simulink model "PID_Controller_ref"  (R2020b)
settings: Solver=ode45  StartTime=0.0  StopTime=0.2  RelTol=1e-3
undefined symbols (not defined in the file or in its folder): Kd, Ki, Kp
settings Model: DataDictionary=DataDictionary.sldd  PacingRate=1000000  Creator=abhin  LastModifiedBy=abhin
settings SolverCC: InitialStep=0.0001  AlgebraicLoopSolver=LineSearch
settings DataIOCC: SaveOutput=off  SaveTime=off

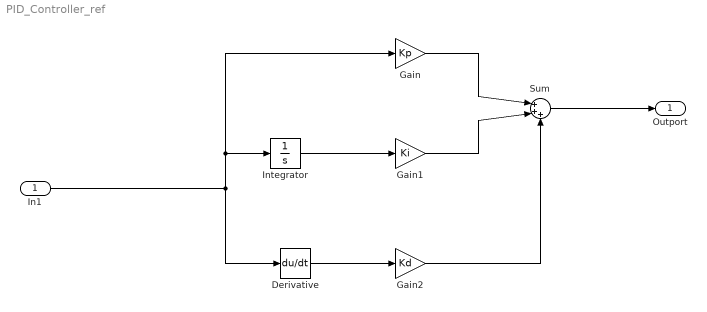
== system PID_Controller_ref ==
  In1 : Inport  OutDataTypeStr=double  PortDimensions=1  SampleTime=0
  Derivative : Derivative
  Gain : Gain  Gain=Kp
  Gain1 : Gain  Gain=Ki
  Gain2 : Gain  Gain=Kd
  Integrator : Integrator
  Sum : Sum  Inputs=|+++
  Outport : Outport  OutDataTypeStr=double  PortDimensions=1  SampleTime=0
  wires:
  Gain2/1 -> Sum/3
  Gain/1 -> Sum/1
  In1/1 -> Gain/1, Integrator/1, Derivative/1
  Gain1/1 -> Sum/2
  Sum/1 -> Outport/1
  Integrator/1 -> Gain1/1
  Derivative/1 -> Gain2/1
